simulink model "HUAUV_UNDERWATER"  (R2018a)
settings: Solver=VariableStepAuto  StartTime=0.0  StopTime=50  MaxStep=0.002  RelTol=1e-3
InitFcn:
  | run('HUAUVInitial.m')
values from neighbouring files (symbols this model uses):
  buoPos =     [HUAUVPARAMETERS.mat]
  coeff =     [HUAUVPARAMETERS.mat]
  g = 9.8    [HUAUVInitial.m]    (also in HUAUVPARAMETERS.mat)
  Jx = 2.365e-2    (= 0.02365)    [HUAUVInitial.m]    (also in HUAUVPARAMETERS.mat)
  Jy = 1.318e-2    (= 0.01318)    [HUAUVInitial.m]    (also in HUAUVPARAMETERS.mat)
  Jz = 1.318e-2    (= 0.01318)    [HUAUVInitial.m]    (also in HUAUVPARAMETERS.mat)
  m = 1.8    [HUAUVInitial.m]    (also in HUAUVPARAMETERS.mat)
  Sx = 0.07*0.15    (= 0.0105)    [HUAUVInitial.m]    (also in HUAUVPARAMETERS.mat)
  Sy = 0.07*0.28    (= 0.0196)    [HUAUVInitial.m]    (also in HUAUVPARAMETERS.mat)
  Sz = 0.15*0.28    (= 0.042)    [HUAUVInitial.m]    (also in HUAUVPARAMETERS.mat)
  V = 1e-3    (= 0.001)    [HUAUVInitial.m]
undefined symbols (not defined in the file or in its folder): rho
libraries: simulink x6, shared6dof x1
settings Model: Creator=MI  LastModifiedBy=MI
settings SolverCC: ZeroCrossAlgorithm=Adaptive
settings DebuggingCC: MaxConsecutiveZCsMsg=none

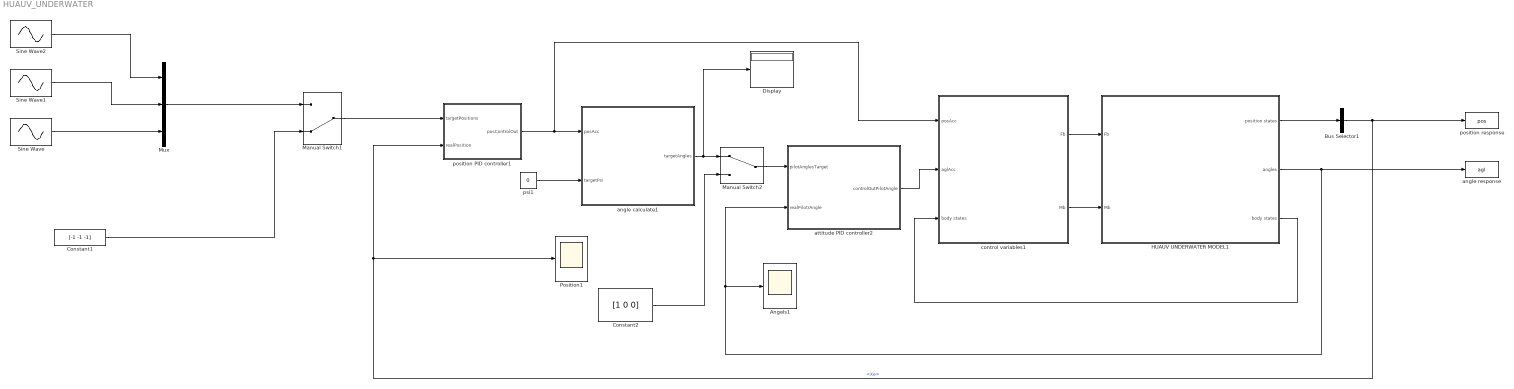
== system HUAUV_UNDERWATER ==
  Angels1 : Scope
  Bus Selector1 : BusSelector  OutputSignals=Xe
  Constant1 : Constant  Value=[-1 -1 -1]
  Constant2 : Constant  Value=[1 0 0]
  Display : Display
  HUAUV UNDERWATER MODEL1 : Subsystem
  Manual Switch1 : ManualSwitch  CurrentSetting=0
  Manual Switch2 : ManualSwitch
  Mux : Mux  Inputs=3
  Position1 : Scope
  Sine Wave : Sin  Bias=-2  Frequency=2  SampleTime=0
  Sine Wave1 : Sin  Frequency=2  Phase=pi/2  SampleTime=0
  Sine Wave2 : Sin  Frequency=2  Phase=pi/3  SampleTime=0
  angle calculate1 : Subsystem
  angle response : ToWorkspace  VariableName=agl  SampleTime=-1
  attitude PID controller2 : Subsystem
  control variables1 : Subsystem
  position PID controller1 : Subsystem
  position response : ToWorkspace  VariableName=pos  SampleTime=-1
  psi1 : Constant  Value=0
  wires:
  Sine Wave/1 -> Mux/3
  Sine Wave1/1 -> Mux/2
  Sine Wave2/1 -> Mux/1
  Mux/1 -> Manual Switch1/1
  Constant1/1 -> Manual Switch1/2
  position PID controller1/1(posControlOut) -> control variables1/1(posAcc), angle calculate1/1(posAcc)
  psi1/1 -> angle calculate1/2(targetPsi)
  Manual Switch2/1 -> attitude PID controller2/1(pilotAnglesTarget)
  angle calculate1/1(targetAngles) -> Display/1, Manual Switch2/1
  Constant2/1 -> Manual Switch2/2
  Manual Switch1/1 -> position PID controller1/1(targetPositions)
  control variables1/2(Mb) -> HUAUV UNDERWATER MODEL1/2(Mb)
  HUAUV UNDERWATER MODEL1/2(angles) -> angle response/1, attitude PID controller2/2(realPilotrAngle), Angels1/1
  HUAUV UNDERWATER MODEL1/1(position states) -> Bus Selector1/1
  HUAUV UNDERWATER MODEL1/3(body states) -> control variables1/3(body states)
  Bus Selector1/1 -> position response/1, position PID controller1/2(realPosition), Position1/1  "<Xe>"
  control variables1/1(Fb) -> HUAUV UNDERWATER MODEL1/1(Fb)
  attitude PID controller2/1(controlOutPilotAngle) -> control variables1/2(aglAcc)

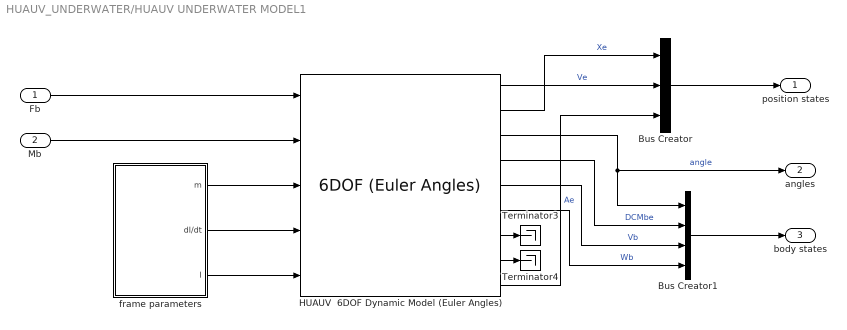
== system HUAUV_UNDERWATER/HUAUV UNDERWATER MODEL1 ==
  Fb : Inport
  Mb : Inport  Port=2
  Bus Creator : BusCreator  Inputs=3
  Bus Creator1 : BusCreator  Inputs=4
  HUAUV  6DOF Dynamic Model (Euler Angles) : shared6dof/6DOF (Euler Angles)  units=Metric (MKS)  mtype=Custom Variable  rep=Euler Angles  xme_0=[0 0 0]  Vm_0=[0 0 0]  eul_0=[0 0 0]  pm_0=[0 0 0]  mass_0=1.0  mass_e=0.5  mass_f=2.0  inertia=eye(3)  inertia_e=eye(3)  inertia_f=2*eye(3)  k_quat=1.0  vre_flag=off  abi_flag=on  aMode=0
      settings: SourceProductBaseCode=AE
  Terminator3 : Terminator
  Terminator4 : Terminator
  frame parameters : Subsystem
  position states : Outport
  angles : Outport  Port=2
  body states : Outport  Port=3
  wires:
  HUAUV  6DOF Dynamic Model (Euler Angles)/2 -> Bus Creator/1  "Xe"
  HUAUV  6DOF Dynamic Model (Euler Angles)/9 -> Bus Creator/3  "Ae"
  frame parameters/1(m) -> HUAUV  6DOF Dynamic Model (Euler Angles)/3
  HUAUV  6DOF Dynamic Model (Euler Angles)/1 -> Bus Creator/2  "Ve"
  HUAUV  6DOF Dynamic Model (Euler Angles)/7 -> Terminator3/1
  HUAUV  6DOF Dynamic Model (Euler Angles)/8 -> Terminator4/1
  Mb/1 -> HUAUV  6DOF Dynamic Model (Euler Angles)/2
  Bus Creator/1 -> position states/1
  frame parameters/2(dI/dt) -> HUAUV  6DOF Dynamic Model (Euler Angles)/4
  frame parameters/3(I) -> HUAUV  6DOF Dynamic Model (Euler Angles)/5
  Fb/1 -> HUAUV  6DOF Dynamic Model (Euler Angles)/1
  HUAUV  6DOF Dynamic Model (Euler Angles)/3 -> angles/1, Bus Creator1/1  "angle"
  Bus Creator1/1 -> body states/1
  HUAUV  6DOF Dynamic Model (Euler Angles)/6 -> Bus Creator1/4  "Wb"
  HUAUV  6DOF Dynamic Model (Euler Angles)/5 -> Bus Creator1/3  "Vb"
  HUAUV  6DOF Dynamic Model (Euler Angles)/4 -> Bus Creator1/2  "DCMbe"

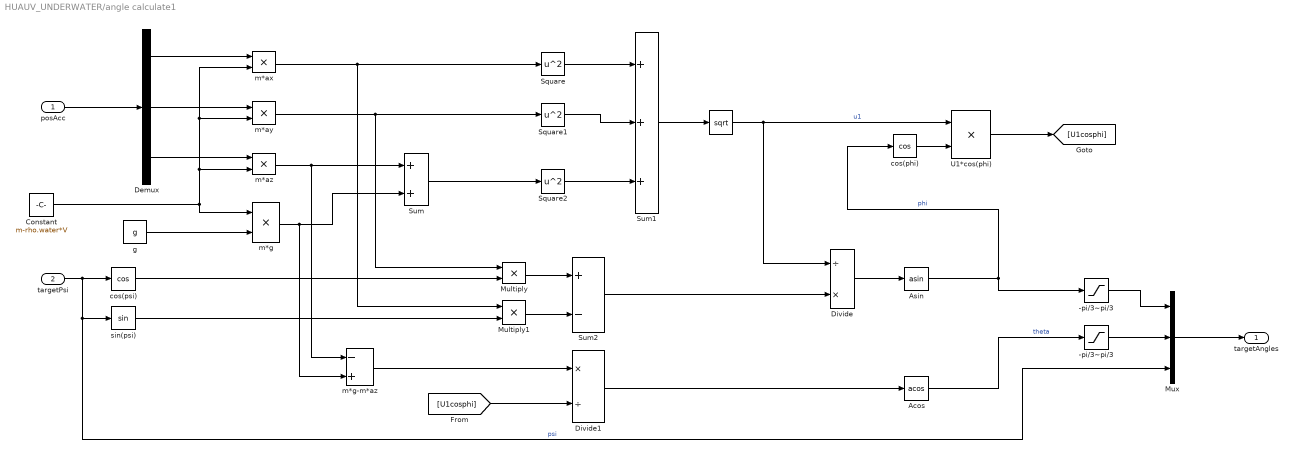
== system HUAUV_UNDERWATER/angle calculate1 ==
  posAcc : Inport
  targetPsi : Inport  Port=2
  " " : Sqrt  SaturateOnIntegerOverflow=on
  -pi/3~pi/3 : Saturate  UpperLimit=pi/3  LowerLimit=-pi/3
  "-pi/3~pi/3  " : Saturate  UpperLimit=pi/3  LowerLimit=-pi/3
  Acos : Trigonometry  Operator=acos
  Asin : Trigonometry  Operator=asin
  Constant : Constant  Value=m-rho.water*V
  Demux : Demux  Outputs=3
  Divide : Product  Inputs=/*
  Divide1 : Product  Inputs=*/
  Multiply : Product
  Multiply1 : Product
  Mux : Mux  Inputs=3
  Square : Math  Operator=square  SaturateOnIntegerOverflow=on
  Square1 : Math  Operator=square  SaturateOnIntegerOverflow=on
  Square2 : Math  Operator=square  SaturateOnIntegerOverflow=on
  Sum : Sum
  Sum1 : Sum  Inputs=+++
  Sum2 : Sum  Inputs=+-
  U1*cos(phi) : Product
  cos(phi) : Trigonometry  Operator=cos
  cos(psi) : Trigonometry  Operator=cos
  g : Constant  Value=g
  m*ax : Product
  m*ay : Product
  m*az : Product
  m*g : Product
  m*g-m*az : Sum  Inputs=-+
  sin(psi) : Trigonometry
  targetAngles : Outport
  wires:
  posAcc/1 -> Demux/1
  Demux/3 -> m*az/1
  Demux/2 -> m*ay/1
  Demux/1 -> m*ax/1
  Constant/1 -> m*g/1, m*ax/2, m*ay/2, m*az/2
  m*ay/1 -> Square1/1, Multiply/1
  m*ax/1 -> Multiply1/1, Square/1
  g/1 -> m*g/2
  m*g/1 -> m*g-m*az/2, Sum/2
  m*az/1 -> m*g-m*az/1, Sum/1
  Sum/1 -> Square2/1
  Square/1 -> Sum1/1
  Square2/1 -> Sum1/3
  Square1/1 -> Sum1/2
  Sum1/1 -> " "/1
  targetPsi/1 -> Mux/3, sin(psi)/1, cos(psi)/1  "psi"
  cos(psi)/1 -> Multiply/2
  sin(psi)/1 -> Multiply1/2
  Multiply1/1 -> Sum2/2
  Multiply/1 -> Sum2/1
  Sum2/1 -> Divide/2
  " "/1 -> Divide/1, U1*cos(phi)/1  "u1"
  Divide/1 -> Asin/1
  Asin/1 -> -pi/3~pi/3/1, cos(phi)/1  "phi"
  Mux/1 -> targetAngles/1
  Acos/1 -> "-pi/3~pi/3  "/1  "theta"
  cos(phi)/1 -> U1*cos(phi)/2
  U1*cos(phi)/1 -> [U1cosphi]
  m*g-m*az/1 -> Divide1/1
  [U1cosphi] -> Divide1/2
  Divide1/1 -> Acos/1
  -pi/3~pi/3/1 -> Mux/1
  "-pi/3~pi/3  "/1 -> Mux/2

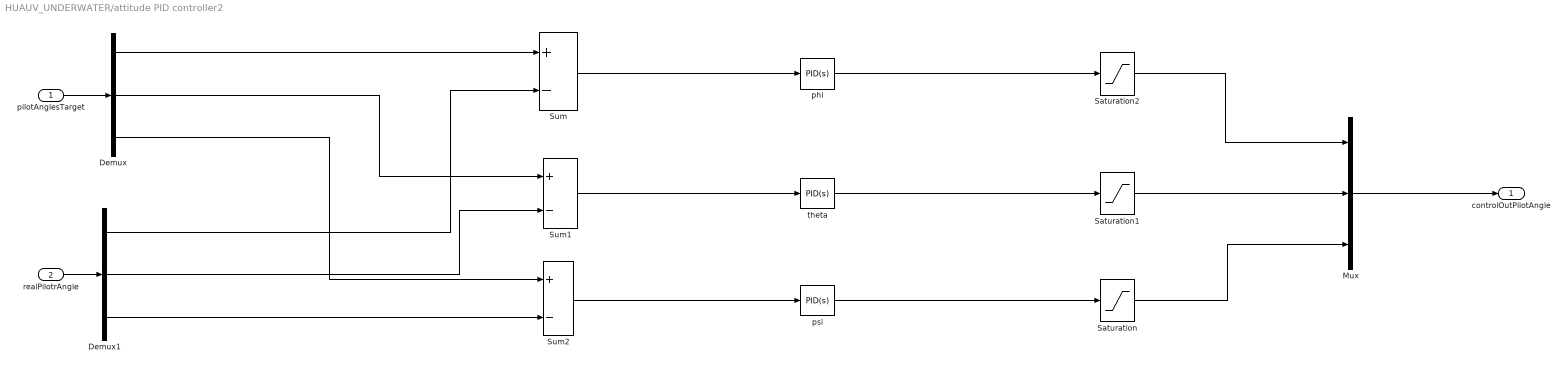
== system HUAUV_UNDERWATER/attitude PID controller2 ==
  pilotAnglesTarget : Inport
  realPilotrAngle : Inport  Port=2
  Demux : Demux  Outputs=3
  Demux1 : Demux  Outputs=3
  Mux : Mux  Inputs=3
  Saturation : Saturate  UpperLimit=80  LowerLimit=-80
  Saturation1 : Saturate  UpperLimit=100  LowerLimit=-100
  Saturation2 : Saturate  UpperLimit=100  LowerLimit=-100
  Sum : Sum  Inputs=+-
  Sum1 : Sum  Inputs=+-
  Sum2 : Sum  Inputs=+-
  phi : simulink/Continuous/PID Controller  Controller=PID  TimeDomain=Continuous-time  SampleTime=-1  IntegratorMethod=Forward Euler  FilterMethod=Forward Euler  Form=Parallel  UseFilter=on  ControllerParametersSource=internal  P=607.007237650316  I=538.5363122748  D=152.017546187089  N=17379.6431323802  InitialConditionSource=internal  InitialConditionForIntegrator=0  InitialConditionForFilter=0  ExternalReset=none  LimitOutput=off  UpperSaturationLimit=inf  LowerSaturationLimit=-inf  LinearizeAsGain=on  AntiWindupMode=none  Kb=1  TrackingMode=off  Kt=1  PParamMin=[]  PParamMax=[]  IParamMin=[]  IParamMax=[]  DParamMin=[]  DParamMax=[]  NParamMin=[]  NParamMax=[]  KbParamMin=[]  KbParamMax=[]  KtParamMin=[]  KtParamMax=[]  POutMin=[]  POutMax=[]  IOutMin=[]  IOutMax=[]  DOutMin=[]  DOutMax=[]  NOutMin=[]  NOutMax=[]  KbOutMin=[]  KbOutMax=[]  KtOutMin=[]  KtOutMax=[]  IntegratorOutMin=[]  IntegratorOutMax=[]  FilterOutMin=[]  FilterOutMax=[]  SumOutMin=[]  SumOutMax=[]  SumI1OutMin=[]  SumI1OutMax=[]  SumI2OutMin=[]  SumI2OutMax=[]  SumI3OutMin=[]  SumI3OutMax=[]  SumDOutMin=[]  SumDOutMax=[]  SaturationOutMin=[]  SaturationOutMax=[]  IntegratorContinuousStateAttributes=''  IntegratorStateMustResolveToSignalObject=off  IntegratorRTWStateStorageClass=Auto  FilterContinuousStateAttributes=''  FilterStateMustResolveToSignalObject=off  FilterRTWStateStorageClass=Auto  DifferentiatorICPrevScaledInput=0  DifferentiatorOutMin=[]  DifferentiatorOutMax=[]  FilterDiffOutCoefMin=[]  FilterDiffOutCoefMax=[]  SumDenOutMin=[]  SumDenOutMax=[]  SumNumOutMin=[]  SumNumOutMax=[]  ReciprocalOutMin=[]  ReciprocalOutMax=[]  DivideOutMin=[]  DivideOutMax=[]  TunerSelectOption=Transfer Function Based (PID Tuner App)
  psi : simulink/Continuous/PID Controller  Controller=PID  TimeDomain=Continuous-time  SampleTime=-1  IntegratorMethod=Forward Euler  FilterMethod=Forward Euler  Form=Parallel  UseFilter=on  ControllerParametersSource=internal  P=604.136885456489  I=534.720062935405  D=151.657955362916  N=17338.473494823  InitialConditionSource=internal  InitialConditionForIntegrator=0  InitialConditionForFilter=0  ExternalReset=none  LimitOutput=off  UpperSaturationLimit=inf  LowerSaturationLimit=-inf  LinearizeAsGain=on  AntiWindupMode=none  Kb=1  TrackingMode=off  Kt=1  PParamMin=[]  PParamMax=[]  IParamMin=[]  IParamMax=[]  DParamMin=[]  DParamMax=[]  NParamMin=[]  NParamMax=[]  KbParamMin=[]  KbParamMax=[]  KtParamMin=[]  KtParamMax=[]  POutMin=[]  POutMax=[]  IOutMin=[]  IOutMax=[]  DOutMin=[]  DOutMax=[]  NOutMin=[]  NOutMax=[]  KbOutMin=[]  KbOutMax=[]  KtOutMin=[]  KtOutMax=[]  IntegratorOutMin=[]  IntegratorOutMax=[]  FilterOutMin=[]  FilterOutMax=[]  SumOutMin=[]  SumOutMax=[]  SumI1OutMin=[]  SumI1OutMax=[]  SumI2OutMin=[]  SumI2OutMax=[]  SumI3OutMin=[]  SumI3OutMax=[]  SumDOutMin=[]  SumDOutMax=[]  SaturationOutMin=[]  SaturationOutMax=[]  IntegratorContinuousStateAttributes=''  IntegratorStateMustResolveToSignalObject=off  IntegratorRTWStateStorageClass=Auto  FilterContinuousStateAttributes=''  FilterStateMustResolveToSignalObject=off  FilterRTWStateStorageClass=Auto  DifferentiatorICPrevScaledInput=0  DifferentiatorOutMin=[]  DifferentiatorOutMax=[]  FilterDiffOutCoefMin=[]  FilterDiffOutCoefMax=[]  SumDenOutMin=[]  SumDenOutMax=[]  SumNumOutMin=[]  SumNumOutMax=[]  ReciprocalOutMin=[]  ReciprocalOutMax=[]  DivideOutMin=[]  DivideOutMax=[]  TunerSelectOption=Transfer Function Based (PID Tuner App)
  theta : simulink/Continuous/PID Controller  Controller=PID  TimeDomain=Continuous-time  SampleTime=-1  IntegratorMethod=Forward Euler  FilterMethod=Forward Euler  Form=Parallel  UseFilter=on  ControllerParametersSource=internal  P=105.144370602587  I=38.8392925143905  D=38.8392925143905  N=7236.10760650948  InitialConditionSource=internal  InitialConditionForIntegrator=0  InitialConditionForFilter=0  ExternalReset=none  LimitOutput=off  UpperSaturationLimit=inf  LowerSaturationLimit=-inf  LinearizeAsGain=on  AntiWindupMode=none  Kb=1  TrackingMode=off  Kt=1  PParamMin=[]  PParamMax=[]  IParamMin=[]  IParamMax=[]  DParamMin=[]  DParamMax=[]  NParamMin=[]  NParamMax=[]  KbParamMin=[]  KbParamMax=[]  KtParamMin=[]  KtParamMax=[]  POutMin=[]  POutMax=[]  IOutMin=[]  IOutMax=[]  DOutMin=[]  DOutMax=[]  NOutMin=[]  NOutMax=[]  KbOutMin=[]  KbOutMax=[]  KtOutMin=[]  KtOutMax=[]  IntegratorOutMin=[]  IntegratorOutMax=[]  FilterOutMin=[]  FilterOutMax=[]  SumOutMin=[]  SumOutMax=[]  SumI1OutMin=[]  SumI1OutMax=[]  SumI2OutMin=[]  SumI2OutMax=[]  SumI3OutMin=[]  SumI3OutMax=[]  SumDOutMin=[]  SumDOutMax=[]  SaturationOutMin=[]  SaturationOutMax=[]  IntegratorContinuousStateAttributes=''  IntegratorStateMustResolveToSignalObject=off  IntegratorRTWStateStorageClass=Auto  FilterContinuousStateAttributes=''  FilterStateMustResolveToSignalObject=off  FilterRTWStateStorageClass=Auto  DifferentiatorICPrevScaledInput=0  DifferentiatorOutMin=[]  DifferentiatorOutMax=[]  FilterDiffOutCoefMin=[]  FilterDiffOutCoefMax=[]  SumDenOutMin=[]  SumDenOutMax=[]  SumNumOutMin=[]  SumNumOutMax=[]  ReciprocalOutMin=[]  ReciprocalOutMax=[]  DivideOutMin=[]  DivideOutMax=[]  TunerSelectOption=Transfer Function Based (PID Tuner App)
  controlOutPilotAngle : Outport
  wires:
  Sum2/1 -> psi/1
  psi/1 -> Saturation/1
  Demux1/2 -> Sum1/2
  phi/1 -> Saturation2/1
  Demux1/1 -> Sum/2
  Demux/2 -> Sum1/1
  Sum/1 -> phi/1
  Demux/3 -> Sum2/1
  Sum1/1 -> theta/1
  Demux1/3 -> Sum2/2
  theta/1 -> Saturation1/1
  Demux/1 -> Sum/1
  pilotAnglesTarget/1 -> Demux/1
  realPilotrAngle/1 -> Demux1/1
  Mux/1 -> controlOutPilotAngle/1
  Saturation/1 -> Mux/3
  Saturation2/1 -> Mux/1
  Saturation1/1 -> Mux/2

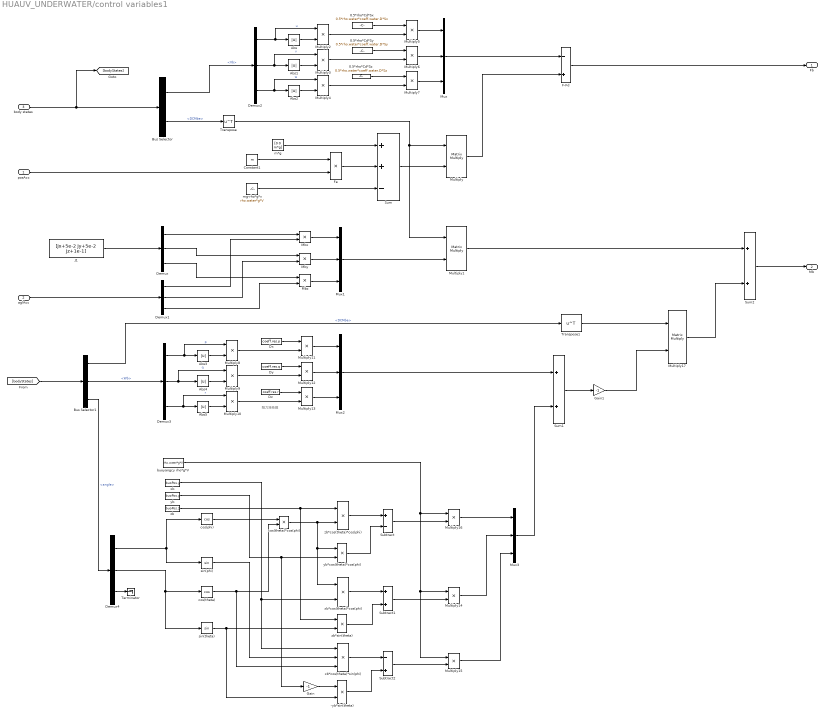
== system HUAUV_UNDERWATER/control variables1 ==
  note: 阻力矩系数
  posAcc : Inport
  aglAcc : Inport  Port=2
  body states : Inport  Port=3
  -yb*sin(theta) : Product
  0.5*rho*Cd*Sx : Constant  Value=0.5*rho.water*coeff.water.D*Sx
  0.5*rho*Cd*Sy : Constant  Value=0.5*rho.water*coeff.water.D*Sy
  0.5*rho*Cd*Sz : Constant  Value=0.5*rho.water*coeff.water.D*Sz
  Abs{,1..5} (6 alike) : Abs
  Bus Selector : BusSelector  OutputSignals=Vb,DCMbe
  Bus Selector1 : BusSelector  OutputSignals=DCMbe,Wb,angle
  Constant1 : Constant  Value=m
  Demux{,1..4} (5 alike) : Demux  Outputs=3
  Dx : Constant  Value=coeff.res.p
  Dy : Constant  Value=coeff.res.q
  Dz : Constant  Value=coeff.res.r
  F-Fd : Sum  Inputs=-+
  Fe : Product
  Gain : Gain  Gain=-1
  Gain1 : Gain  Gain=-1
  J1 : Constant  Value=[Jx+5e-2 Jy+5e-2 Jz+1e-1]
  Mbx : Product
  Mby : Product
  Mbz : Product
  Multiply : Product  Multiplication=Matrix(*)
  Multiply1 : Product  Multiplication=Matrix(*)
  Multiply{2..16} (15 alike) : Product
  Multiply17 : Product  Multiplication=Matrix(*)
  Mux{,1..3} (4 alike) : Mux  Inputs=3
  Subtract : Sum  Inputs=+-
  Subtract1 : Sum
  Subtract2 : Sum  Inputs=-+
  Sum : Sum  Inputs=++-
  Sum1 : Sum
  Sum2 : Sum
  Terminator : Terminator
  Transpose : Math  Operator=transpose  SaturateOnIntegerOverflow=on
  Transpose1 : Math  Operator=transpose  SaturateOnIntegerOverflow=on
  buoyangcy rho*g*V : Constant  Value=rho.water*g*V
  cos(phi) : Trigonometry  Operator=cos
  cos(theta) : Trigonometry  Operator=cos
  cos(theta)*cos(phi) : Product
  m*g : Constant  Value=[0 0 m*g]
  mg-rho*g*v : Constant  Value=rho.water*g*V
  sin(phi) : Trigonometry
  sin(theta) : Trigonometry
  xb : Constant  Value=buoPos.y
  xb*cos(theta)*cos(phi) : Product
  xb*cos(theta)*sin(phi) : Product  Inputs=3
  yb : Constant  Value=buoPos.y
  yb*cos(theta)*cos(phi) : Product
  zb : Constant  Value=buoPos.z
  zb*cos(theta)*cos(phi) : Product
  zb*sin(theta) : Product
  Fb : Outport
  Mb : Outport  Port=2
  wires:
  Demux/3 -> Mbz/1
  Demux1/2 -> Mby/2
  Demux/2 -> Mby/1
  Demux/1 -> Mbx/1
  Demux1/3 -> Mbz/2
  Demux1/1 -> Mbx/2
  aglAcc/1 -> Demux1/1
  J1/1 -> Demux/1
  Mby/1 -> Mux1/2
  Mbx/1 -> Mux1/1
  Mbz/1 -> Mux1/3
  Fe/1 -> Sum/2
  m*g/1 -> Sum/1
  Constant1/1 -> Fe/1
  posAcc/1 -> Fe/2
  Sum/1 -> Multiply/2
  Mux1/1 -> Multiply1/2
  mg-rho*g*v/1 -> Sum/3
  Bus Selector/2 -> Transpose/1  "<DCMbe>"
  Transpose/1 -> Multiply/1, Multiply1/1
  Multiply3/1 -> Multiply6/2
  Abs1/1 -> Multiply3/2
  Demux2/2 -> Multiply3/1, Abs1/1  "v"
  0.5*rho*Cd*Sz/1 -> Multiply7/1
  Abs/1 -> Multiply2/2
  Abs2/1 -> Multiply4/2
  Demux2/1 -> Multiply2/1, Abs/1  "u"
  Demux2/3 -> Abs2/1, Multiply4/1  "w"
  0.5*rho*Cd*Sy/1 -> Multiply6/1
  Multiply2/1 -> Multiply5/2
  Multiply4/1 -> Multiply7/2
  0.5*rho*Cd*Sx/1 -> Multiply5/1
  Multiply6/1 -> Mux/2
  Multiply5/1 -> Mux/1
  Multiply7/1 -> Mux/3
  Mux/1 -> F-Fd/1
  Multiply/1 -> F-Fd/2
  F-Fd/1 -> Fb/1
  Bus Selector/1 -> Demux2/1  "<Vb>"
  body states/1 -> [bodyStates], Bus Selector/1
  Dx/1 -> Multiply11/1
  Demux3/2 -> Abs4/1, Multiply9/1  "q"
  Bus Selector1/2 -> Demux3/1  "<Wb>"
  Demux3/1 -> Multiply8/1, Abs3/1  "p"
  Dy/1 -> Multiply12/1
  Multiply9/1 -> Multiply12/2
  Abs4/1 -> Multiply9/2
  Abs5/1 -> Multiply10/2
  Demux3/3 -> Abs5/1, Multiply10/1  "r"
  Abs3/1 -> Multiply8/2
  Multiply8/1 -> Multiply11/2
  Multiply10/1 -> Multiply13/2
  Dz/1 -> Multiply13/1
  [bodyStates] -> Bus Selector1/1
  Multiply13/1 -> Mux2/3
  Multiply12/1 -> Mux2/2
  Multiply11/1 -> Mux2/1
  sin(theta)/1 -> -yb*sin(theta)/2, zb*sin(theta)/2
  Subtract1/1 -> Multiply14/2
  xb/1 -> xb*cos(theta)*sin(phi)/1, xb*cos(theta)*cos(phi)/2
  Gain/1 -> -yb*sin(theta)/1
  buoyangcy rho*g*V/1 -> Multiply15/1, Multiply14/1, Multiply16/1
  Subtract2/1 -> Multiply15/2
  yb/1 -> Gain/1, yb*cos(theta)*cos(phi)/2
  Demux4/1 -> cos(phi)/1, sin(phi)/1
  Demux4/2 -> sin(theta)/1, cos(theta)/1
  cos(theta)*cos(phi)/1 -> zb*cos(theta)*cos(phi)/2, xb*cos(theta)*cos(phi)/1, yb*cos(theta)*cos(phi)/1
  zb*sin(theta)/1 -> Subtract1/2
  sin(phi)/1 -> xb*cos(theta)*sin(phi)/2
  zb/1 -> zb*sin(theta)/1, zb*cos(theta)*cos(phi)/1
  zb*cos(theta)*cos(phi)/1 -> Subtract/1
  yb*cos(theta)*cos(phi)/1 -> Subtract/2
  xb*cos(theta)*sin(phi)/1 -> Subtract2/1
  Subtract/1 -> Multiply16/2
  -yb*sin(theta)/1 -> Subtract2/2
  cos(phi)/1 -> cos(theta)*cos(phi)/1
  xb*cos(theta)*cos(phi)/1 -> Subtract1/1
  cos(theta)/1 -> xb*cos(theta)*sin(phi)/3, cos(theta)*cos(phi)/2
  Bus Selector1/3 -> Demux4/1  "<angle>"
  Demux4/3 -> Terminator/1
  Multiply14/1 -> Mux3/2
  Multiply16/1 -> Mux3/1
  Multiply15/1 -> Mux3/3
  Mux2/1 -> Sum1/1
  Mux3/1 -> Sum1/2
  Sum1/1 -> Gain1/1
  Bus Selector1/1 -> Transpose1/1  "<DCMbe>"
  Transpose1/1 -> Multiply17/1
  Gain1/1 -> Multiply17/2
  Multiply1/1 -> Sum2/1
  Multiply17/1 -> Sum2/2
  Sum2/1 -> Mb/1

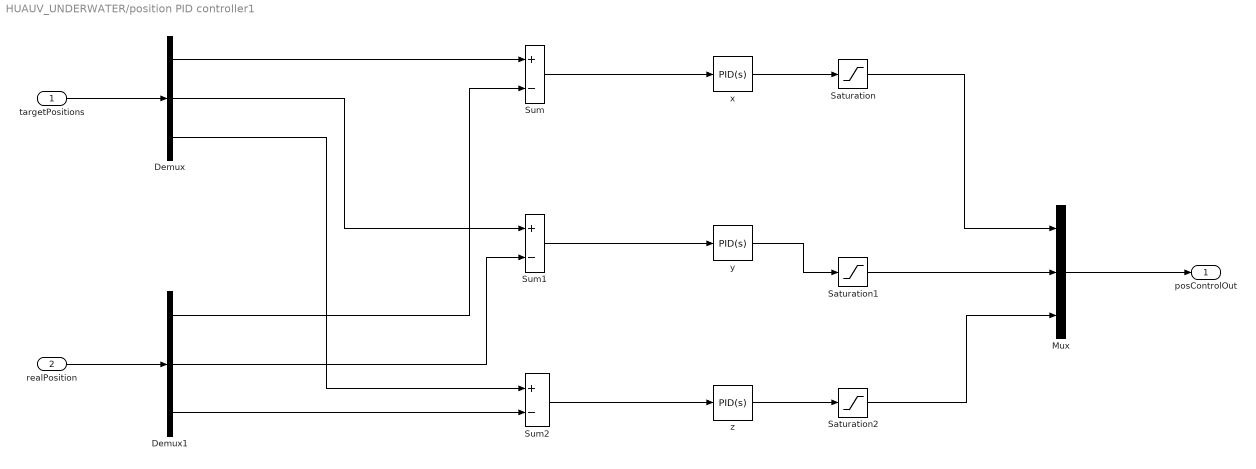
== system HUAUV_UNDERWATER/position PID controller1 ==
  targetPositions : Inport
  realPosition : Inport  Port=2
  Demux : Demux  Outputs=3
  Demux1 : Demux  Outputs=3
  Mux : Mux  Inputs=3
  Saturation : Saturate  UpperLimit=100  LowerLimit=-100
  Saturation1 : Saturate  UpperLimit=100  LowerLimit=-100
  Saturation2 : Saturate  UpperLimit=200  LowerLimit=-200
  Sum : Sum  Inputs=+-
  Sum1 : Sum  Inputs=+-
  Sum2 : Sum  Inputs=+-
  x : simulink/Continuous/PID Controller  Controller=PID  TimeDomain=Continuous-time  SampleTime=-1  IntegratorMethod=Forward Euler  FilterMethod=Forward Euler  Form=Parallel  UseFilter=on  ControllerParametersSource=internal  P=150  I=70  D=80  N=9099.36023942606  InitialConditionSource=internal  InitialConditionForIntegrator=0  InitialConditionForFilter=0  ExternalReset=none  LimitOutput=off  UpperSaturationLimit=inf  LowerSaturationLimit=-inf  LinearizeAsGain=on  AntiWindupMode=none  Kb=1  TrackingMode=off  Kt=1  PParamMin=[]  PParamMax=[]  IParamMin=[]  IParamMax=[]  DParamMin=[]  DParamMax=[]  NParamMin=[]  NParamMax=[]  KbParamMin=[]  KbParamMax=[]  KtParamMin=[]  KtParamMax=[]  POutMin=[]  POutMax=[]  IOutMin=[]  IOutMax=[]  DOutMin=[]  DOutMax=[]  NOutMin=[]  NOutMax=[]  KbOutMin=[]  KbOutMax=[]  KtOutMin=[]  KtOutMax=[]  IntegratorOutMin=[]  IntegratorOutMax=[]  FilterOutMin=[]  FilterOutMax=[]  SumOutMin=[]  SumOutMax=[]  SumI1OutMin=[]  SumI1OutMax=[]  SumI2OutMin=[]  SumI2OutMax=[]  SumI3OutMin=[]  SumI3OutMax=[]  SumDOutMin=[]  SumDOutMax=[]  SaturationOutMin=[]  SaturationOutMax=[]  IntegratorContinuousStateAttributes=''  IntegratorStateMustResolveToSignalObject=off  IntegratorRTWStateStorageClass=Auto  FilterContinuousStateAttributes=''  FilterStateMustResolveToSignalObject=off  FilterRTWStateStorageClass=Auto  DifferentiatorICPrevScaledInput=0  DifferentiatorOutMin=[]  DifferentiatorOutMax=[]  FilterDiffOutCoefMin=[]  FilterDiffOutCoefMax=[]  SumDenOutMin=[]  SumDenOutMax=[]  SumNumOutMin=[]  SumNumOutMax=[]  ReciprocalOutMin=[]  ReciprocalOutMax=[]  DivideOutMin=[]  DivideOutMax=[]  TunerSelectOption=Transfer Function Based (PID Tuner App)
  y : simulink/Continuous/PID Controller  Controller=PID  TimeDomain=Continuous-time  SampleTime=-1  IntegratorMethod=Forward Euler  FilterMethod=Forward Euler  Form=Parallel  UseFilter=on  ControllerParametersSource=internal  P=36.8420392063011  I=3.4  D=51.7115453208585  N=1442.15140992177  InitialConditionSource=internal  InitialConditionForIntegrator=0  InitialConditionForFilter=0  ExternalReset=none  LimitOutput=off  UpperSaturationLimit=inf  LowerSaturationLimit=-inf  LinearizeAsGain=on  AntiWindupMode=none  Kb=1  TrackingMode=off  Kt=1  PParamMin=[]  PParamMax=[]  IParamMin=[]  IParamMax=[]  DParamMin=[]  DParamMax=[]  NParamMin=[]  NParamMax=[]  KbParamMin=[]  KbParamMax=[]  KtParamMin=[]  KtParamMax=[]  POutMin=[]  POutMax=[]  IOutMin=[]  IOutMax=[]  DOutMin=[]  DOutMax=[]  NOutMin=[]  NOutMax=[]  KbOutMin=[]  KbOutMax=[]  KtOutMin=[]  KtOutMax=[]  IntegratorOutMin=[]  IntegratorOutMax=[]  FilterOutMin=[]  FilterOutMax=[]  SumOutMin=[]  SumOutMax=[]  SumI1OutMin=[]  SumI1OutMax=[]  SumI2OutMin=[]  SumI2OutMax=[]  SumI3OutMin=[]  SumI3OutMax=[]  SumDOutMin=[]  SumDOutMax=[]  SaturationOutMin=[]  SaturationOutMax=[]  IntegratorContinuousStateAttributes=''  IntegratorStateMustResolveToSignalObject=off  IntegratorRTWStateStorageClass=Auto  FilterContinuousStateAttributes=''  FilterStateMustResolveToSignalObject=off  FilterRTWStateStorageClass=Auto  DifferentiatorICPrevScaledInput=0  DifferentiatorOutMin=[]  DifferentiatorOutMax=[]  FilterDiffOutCoefMin=[]  FilterDiffOutCoefMax=[]  SumDenOutMin=[]  SumDenOutMax=[]  SumNumOutMin=[]  SumNumOutMax=[]  ReciprocalOutMin=[]  ReciprocalOutMax=[]  DivideOutMin=[]  DivideOutMax=[]  TunerSelectOption=Transfer Function Based (PID Tuner App)
  z : simulink/Continuous/PID Controller  Controller=PID  TimeDomain=Continuous-time  SampleTime=-1  IntegratorMethod=Forward Euler  FilterMethod=Forward Euler  Form=Parallel  UseFilter=on  ControllerParametersSource=internal  P=59  I=10  D=71.2928934671724  N=3622.5205587649  InitialConditionSource=internal  InitialConditionForIntegrator=0  InitialConditionForFilter=0  ExternalReset=none  LimitOutput=off  UpperSaturationLimit=inf  LowerSaturationLimit=-inf  LinearizeAsGain=on  AntiWindupMode=none  Kb=1  TrackingMode=off  Kt=1  PParamMin=[]  PParamMax=[]  IParamMin=[]  IParamMax=[]  DParamMin=[]  DParamMax=[]  NParamMin=[]  NParamMax=[]  KbParamMin=[]  KbParamMax=[]  KtParamMin=[]  KtParamMax=[]  POutMin=[]  POutMax=[]  IOutMin=[]  IOutMax=[]  DOutMin=[]  DOutMax=[]  NOutMin=[]  NOutMax=[]  KbOutMin=[]  KbOutMax=[]  KtOutMin=[]  KtOutMax=[]  IntegratorOutMin=[]  IntegratorOutMax=[]  FilterOutMin=[]  FilterOutMax=[]  SumOutMin=[]  SumOutMax=[]  SumI1OutMin=[]  SumI1OutMax=[]  SumI2OutMin=[]  SumI2OutMax=[]  SumI3OutMin=[]  SumI3OutMax=[]  SumDOutMin=[]  SumDOutMax=[]  SaturationOutMin=[]  SaturationOutMax=[]  IntegratorContinuousStateAttributes=''  IntegratorStateMustResolveToSignalObject=off  IntegratorRTWStateStorageClass=Auto  FilterContinuousStateAttributes=''  FilterStateMustResolveToSignalObject=off  FilterRTWStateStorageClass=Auto  DifferentiatorICPrevScaledInput=0  DifferentiatorOutMin=[]  DifferentiatorOutMax=[]  FilterDiffOutCoefMin=[]  FilterDiffOutCoefMax=[]  SumDenOutMin=[]  SumDenOutMax=[]  SumNumOutMin=[]  SumNumOutMax=[]  ReciprocalOutMin=[]  ReciprocalOutMax=[]  DivideOutMin=[]  DivideOutMax=[]  TunerSelectOption=Transfer Function Based (PID Tuner App)
  posControlOut : Outport
  wires:
  Sum1/1 -> y/1
  y/1 -> Saturation1/1
  Demux1/2 -> Sum1/2
  Demux/3 -> Sum2/1
  Demux/2 -> Sum1/1
  Demux/1 -> Sum/1
  Sum/1 -> x/1
  z/1 -> Saturation2/1
  Sum2/1 -> z/1
  Demux1/3 -> Sum2/2
  targetPositions/1 -> Demux/1
  realPosition/1 -> Demux1/1
  Mux/1 -> posControlOut/1
  x/1 -> Saturation/1
  Saturation/1 -> Mux/1
  Saturation1/1 -> Mux/2
  Saturation2/1 -> Mux/3
  Demux1/1 -> Sum/2

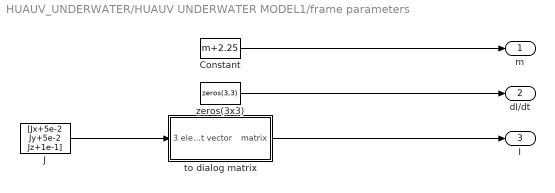
== system HUAUV_UNDERWATER/HUAUV UNDERWATER MODEL1/frame parameters ==
  Constant : Constant  Value=m+2.25
  J : Constant  Value=[Jx+5e-2 Jy+5e-2 Jz+1e-1]
  to dialog matrix : Subsystem
  zeros(3x3) : Constant  Value=zeros(3,3)
  m : Outport
  dI/dt : Outport  Port=2
  I : Outport  Port=3
  wires:
  J/1 -> to dialog matrix/1(3 element vector)
  zeros(3x3)/1 -> dI/dt/1
  Constant/1 -> m/1
  to dialog matrix/1(matrix) -> I/1

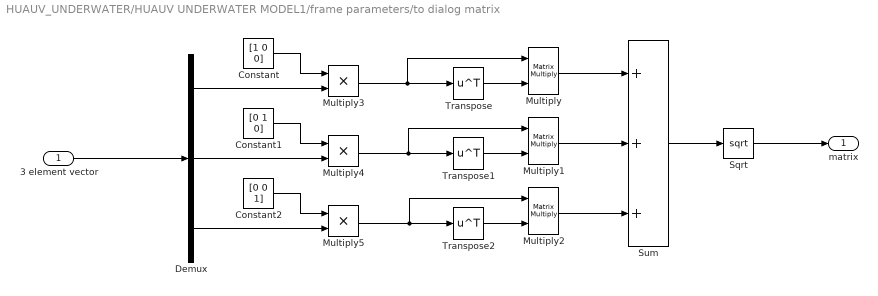
== system HUAUV_UNDERWATER/HUAUV UNDERWATER MODEL1/frame parameters/to dialog matrix ==
  3 element vector : Inport
  Constant : Constant  Value=[1 0 0]
  Constant1 : Constant  Value=[0 1 0]
  Constant2 : Constant  Value=[0 0 1]
  Demux : Demux  Outputs=3
  Multiply : Product  Multiplication=Matrix(*)
  Multiply1 : Product  Multiplication=Matrix(*)
  Multiply2 : Product  Multiplication=Matrix(*)
  Multiply3 : Product
  Multiply4 : Product
  Multiply5 : Product
  Sqrt : Sqrt  SaturateOnIntegerOverflow=on
  Sum : Sum  Inputs=+++
  Transpose : Math  Operator=transpose  SaturateOnIntegerOverflow=on
  Transpose1 : Math  Operator=transpose  SaturateOnIntegerOverflow=on
  Transpose2 : Math  Operator=transpose  SaturateOnIntegerOverflow=on
  matrix : Outport
  wires:
  Sum/1 -> Sqrt/1
  3 element vector/1 -> Demux/1
  Multiply1/1 -> Sum/2
  Multiply/1 -> Sum/1
  Multiply2/1 -> Sum/3
  Demux/1 -> Multiply3/2
  Demux/2 -> Multiply4/2
  Demux/3 -> Multiply5/2
  Constant/1 -> Multiply3/1
  Multiply3/1 -> Multiply/1, Transpose/1
  Constant1/1 -> Multiply4/1
  Constant2/1 -> Multiply5/1
  Multiply4/1 -> Multiply1/1, Transpose1/1
  Transpose/1 -> Multiply/2
  Transpose1/1 -> Multiply1/2
  Transpose2/1 -> Multiply2/2
  Multiply5/1 -> Transpose2/1, Multiply2/1
  Sqrt/1 -> matrix/1
